simulink model "DC_gen_DCBUCK"  (R2025a)
settings: Solver=VariableStepAuto  StartTime=0.0  StopTime=10.0  RelTol=1e-3
undefined symbols (not defined in the file): Grid_DCop_DCBUCK, Sb
settings Model: Creator=atomas  LastModifiedBy=atomas

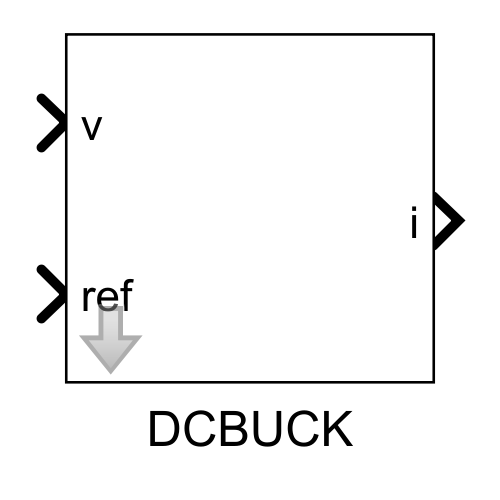
[thumbnail: Simulink's stored preview of the top-level diagram]
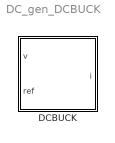
== system DC_gen_DCBUCK ==
  DCBUCK : Subsystem
      mask init:
      | mdlWks = get_param(bdroot,'ModelWorkspace'); % Get the model workspace
      | block_name = get_param(gcb,'Name');
      | try
      |     bvarname = get_param(get_param(get_param(...
      |         gcb, 'Parent'), 'Parent'), 'bvarname');
      |     DC = mdlWks.getVariable([bvarname 'DC']);
      |     block_buses = DC.([block_name 's_buses']);
      |     block_Pg = DC.([block_name 's_Pg']);
      |     block_toM = DC.([block_name 's_toM']);
      | catch ME % block in initialisation
      |     %errordlg(ME.message)
      |     try
      |         DC = mdlWks.getVariable('DC');
      |         block_buses = 1:length(DC.([block_name 's_buses']));
      |         block_Pg = DC.([block_name 's_Pg']);
      |         block_toM = eye(length(block_buses));
      |     catch ME
      |         %errordlg(ME.message)
      |     end
      | end

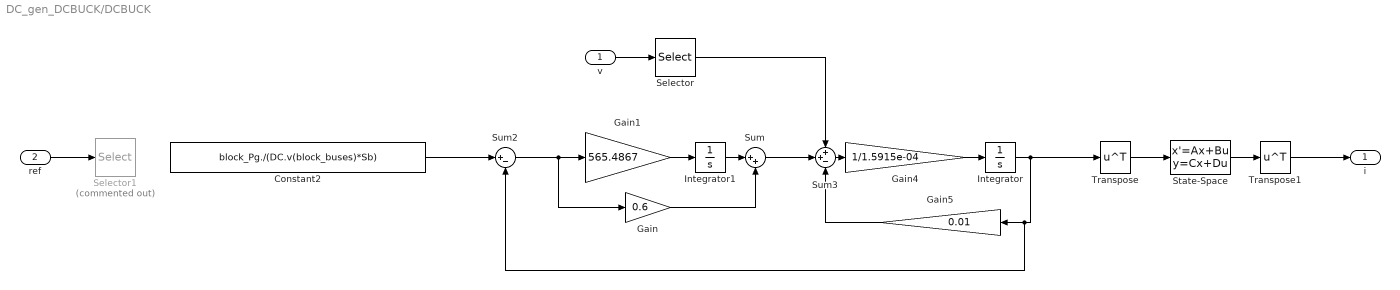
== system DC_gen_DCBUCK/DCBUCK ==
  v : Inport
  ref : Inport  Port=2
  Constant2 : Constant  Value=block_Pg./(DC.v(block_buses)*Sb)  VectorParams1D=off
  Gain : Gain  Gain=0.6
  Gain1 : Gain  Gain=565.4867
  Gain4 : Gain  Gain=1/1.5915e-04
  Gain5 : Gain  Gain=0.01
  Integrator : Integrator  InitialCondition=Grid_DCop_DCBUCK.op.States(1).x'
  Integrator1 : Integrator  InitialCondition=Grid_DCop_DCBUCK.op.States(2).x'
  Selector : Selector  InputPortWidth=DC.Nbuses  IndexOptions=Index vector (dialog)  Indices=block_buses  OutputSizes=1
  Selector1 : Selector  Commented=on  InputPortWidth=3  IndexOptions=Index vector (dialog)  Indices=[1 3]  OutputSizes=1
  State-Space : StateSpace  A=[]  B=[]  C=[]  D=block_toM  InitialCondition=0  ParameterTunability=Optimized
  Sum : Sum  Inputs=|++
  Sum2 : Sum  Inputs=|+-
  Sum3 : Sum  Inputs=++-
  Transpose : Math  Operator=transpose
  Transpose1 : Math  Operator=transpose
  i : Outport
  wires:
  State-Space/1 -> Transpose1/1
  Integrator/1 -> Sum2/2, Gain5/1, Transpose/1
  Transpose/1 -> State-Space/1
  Gain1/1 -> Integrator1/1
  Sum/1 -> Sum3/2
  Gain/1 -> Sum/2
  Integrator1/1 -> Sum/1
  Gain4/1 -> Integrator/1
  Sum2/1 -> Gain1/1, Gain/1
  Transpose1/1 -> i/1
  Sum3/1 -> Gain4/1
  Constant2/1 -> Sum2/1
  ref/1 -> Selector1/1
  v/1 -> Selector/1
  Selector/1 -> Sum3/1
  Gain5/1 -> Sum3/3
